simulink model "template"  (Simulink 5.0)
settings: Solver=ode45  StartTime=0.0  StopTime=10.0  RelTol=1e-3
libraries: cmlib x4
settings Model: LastModifiedBy=ansgar  ExtModeTrigMode=oneshot  ExtModeArmWhenConnect=off  LimitDataPoints=off  BlockReductionOpt=off  BooleanDataType=off

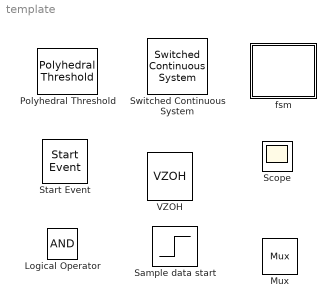
== system template ==
  Logical Operator : Logic
  Mux : Mux  Inputs=2
  Polyhedral Threshold : cmlib/Polyhedral Threshold  polyhedron=floor
  Sample data start : Step  SampleTime=1
  Scope : Scope
      settings: TickLabels=on  DataFormat=Array
  Start Event : cmlib/Start Event  steptime=1  initval=0  finival=1  sampletime=0  interpret=on  enable=on
  Switched Continuous System : cmlib/Switched Continuous System  AncestorBlock=cmlib/Switched Continuous System  nx=1  use_sd=off  nup=[]  nz=[]  use_reset=on  nu=1  x0=1  ICS=linearcon  AR=linearcon  use_param=off  p0=[]  PaCs=[]
  VZOH : cmlib/VZOH  theta=phase  period=period  jitter=jitter
  fsm : Stateflow chart

== stateflow chart fsm ==
